simulink library "halout"  (R2021b)
settings: Solver=VariableStepAuto  StartTime=0.0  StopTime=10.0  RelTol=1e-3
undefined symbols (not defined in the file): C_TASK_5MS_S, FALSE, KHAL_CAN1FD1APS3E2E_flg, KHAL_CAN1FD1APS3TxReq_flg, KHAL_CAN1FD1VCU2E2E_flg, KHAL_CAN1FD1VCU2TxReq_flg, KHAL_CAN1FD1VCU3E2E_flg, KHAL_CAN1FD1VCU3TxReq_flg, KHAL_CAN1TxReq_flg, KHAL_CAN1VMCFCM1E2E_flg, KHAL_CAN1VMCFCM1TxReq_flg, KHAL_CAN2TxReq_flg, KHAL_CAN3FD3VCU1toNIDECTxReq_flg, KHAL_CAN3FD3VCU1TxReq_flg, KHAL_CAN3FD3VCU2E2E_flg, KHAL_CAN3FD3VCU2toNIDECE2E_flg, KHAL_CAN3FD3VCU2toNIDECTxReq_flg, KHAL_CAN3FD3VCU2TxReq_flg, KHAL_CAN3TxReq_flg, KHAL_CAN4FD4CE1000E2E_flg, KHAL_CAN4FD4CE1000TxReq_flg, KHAL_CAN4TxReq_flg, KHAL_CAN5TxReq_flg, KHAL_CAN6FD6APS3E2E_flg, KHAL_CAN6FD6APS3TxReq_flg, KHAL_CAN6FD6VCU2E2E_flg, KHAL_CAN6FD6VCU2TxReq_flg, KHAL_CAN6TxReq_flg, ONE_INT, TRUE, ZERO_INT
libraries: FVT_lib x549, simulink x244
(part 11 of 27)

== system halout/HAL_OUT/CAN4/FD4_CE100_0_Tx ==
  TxReq : Inport
  BSCP_outputs : Inport  Port=2  OutDataTypeStr=Bus: BSCP_outputs
  BOUTP_outputs : Inport  Port=3  OutDataTypeStr=Bus: BOUTP_outputs
  Chart : Stateflow chart  TreatAsAtomicUnit=on
  Constant : Constant  Value=C_TASK_5MS_S
  Constant3 : Constant  Value=CycleTime
  Data Type Conversion : DataTypeConversion  OutDataTypeStr=uint16
  Data Type Conversion1 : DataTypeConversion  OutDataTypeStr=uint8
  Divide : Product  Inputs=*/
  Gain : Gain  Gain=0.001
  Ground{,1..19} (20 alike) : Ground
  OR : Logic  Operator=OR  Inputs=77  AllPortsSameDT=off  OutDataTypeStr=boolean
  bus_selector : BusSelector  OutputSignals=VOUTP_APSStaSys_enum
  bus_selector1 : BusSelector  OutputSignals=VOUTP_AllDoorSW_flg
  bus_selector10 : BusSelector  OutputSignals=VOUTP_DKCAuthSta_enum
  bus_selector11 : BusSelector  OutputSignals=VOUTP_Dimmer_pct
  bus_selector12 : BusSelector  OutputSignals=VOUTP_DimmerEN_flg
  bus_selector13 : BusSelector  OutputSignals=VOUTP_DoorLockIND_flg
  bus_selector14 : BusSelector  OutputSignals=VOUTP_DrDoorSW_flg
  bus_selector15 : BusSelector  OutputSignals=VOUTP_DrSeatSta_enum
  bus_selector16 : BusSelector  OutputSignals=VOUTP_EquivAccPedalSWSta_flg
  bus_selector17 : BusSelector  OutputSignals=VOUTP_FrChargingDoorCtrl_enum
  bus_selector18 : BusSelector  OutputSignals=VOUTP_FrWiperH_flg
  bus_selector19 : BusSelector  OutputSignals=VOUTP_FrWiperL_flg
  bus_selector2 : BusSelector  OutputSignals=VOUTP_AntitheftSeatFlod_flg
  bus_selector20 : BusSelector  OutputSignals=VOUTP_HBeam_flg
  bus_selector21 : BusSelector  OutputSignals=VOUTP_HBeamADB_flg
  bus_selector22 : BusSelector  OutputSignals=VOUTP_HazardSW_flg
  bus_selector23 : BusSelector  OutputSignals=VOUTP_HoodSW_flg
  bus_selector24 : BusSelector  OutputSignals=VOUTP_HornCtrl_flg
  bus_selector25 : BusSelector  OutputSignals=VOUTP_LBSD_flg
  bus_selector26 : BusSelector  OutputSignals=VOUTP_LDRL_flg
  bus_selector27 : BusSelector  OutputSignals=VOUTP_LTurnLP_flg
  bus_selector28 : BusSelector  OutputSignals=VOUTP_LBeam_flg
  bus_selector29 : BusSelector  OutputSignals=VOUTP_LampPwr_flg
  bus_selector3 : BusSelector  OutputSignals=VOUTP_AntitheftSta_enum
  bus_selector30 : BusSelector  OutputSignals=VOUTP_LockSetting_flg
  bus_selector31 : BusSelector  OutputSignals=VOUTP_MSACtrlSta_enum
  bus_selector32 : BusSelector  OutputSignals=VOUTP_MirrorCtrl_enum
  bus_selector33 : BusSelector  OutputSignals=VOUTP_MirrorDefog_flg
  bus_selector34 : BusSelector  OutputSignals=VOUTP_PosLamp_flg
  bus_selector35 : BusSelector  OutputSignals=VOUTP_PsDoorSW_flg
  bus_selector36 : BusSelector  OutputSignals=VOUTP_PowerSta_enum
  bus_selector37 : BusSelector  OutputSignals=VOUTP_RBSD_flg
  bus_selector38 : BusSelector  OutputSignals=VOUTP_RDRL_flg
  bus_selector39 : BusSelector  OutputSignals=VOUTP_RLDoorSW_flg
  bus_selector4 : BusSelector  OutputSignals=VOUTP_BCMDoorLockSta_flg
  bus_selector40 : BusSelector  OutputSignals=VOUTP_RRDoorSW_flg
  bus_selector41 : BusSelector  OutputSignals=VOUTP_RTurnLP_flg
  bus_selector42 : BusSelector  OutputSignals=VOUTP_ReBrakeLPReq_flg
  bus_selector43 : BusSelector  OutputSignals=VOUTP_ReverseLamp_flg
  bus_selector44 : BusSelector  OutputSignals=VOUTP_RoomLampH_flg
  bus_selector45 : BusSelector  OutputSignals=VOUTP_RoomLampL_flg
  bus_selector46 : BusSelector  OutputSignals=VOUTP_RrChargingDoorCtrl_enum
  bus_selector47 : BusSelector  OutputSignals=VOUTP_RrDefog_flg
  bus_selector48 : BusSelector  OutputSignals=VOUTP_RrFogLamp_flg
  bus_selector49 : BusSelector  OutputSignals=VOUTP_RrWiper_flg
  bus_selector5 : BusSelector  OutputSignals=VOUTP_BrakeLamp_flg
  bus_selector50 : BusSelector  OutputSignals=VOUTP_ShiftGearPosn_enum
  bus_selector51 : BusSelector  OutputSignals=VOUTP_TailgateHDSW_flg
  bus_selector52 : BusSelector  OutputSignals=VOUTP_TailgateRemote_enum
  bus_selector53 : BusSelector  OutputSignals=VOUTP_TailgateSW_flg
  bus_selector54 : BusSelector  OutputSignals=VOUTP_TrunkRel_flg
  bus_selector55 : BusSelector  OutputSignals=VOUTP_WasherCtrl_enum
  bus_selector56 : BusSelector  OutputSignals=VOUTP_WiperFixMode_flg
  bus_selector6 : BusSelector  OutputSignals=VOUTP_CCCtrlSta_enum
  bus_selector7 : BusSelector  OutputSignals=VOUTP_CTDCtrl_enum
  bus_selector8 : BusSelector  OutputSignals=VOUTP_CTDLockSW_flg
  bus_selector9 : BusSelector  OutputSignals=VOUTP_CrashDetd_flg
  convert_out : FVT_lib/hal/convert_out  gain=1  offset=0
  detect_change{,1..56} (57 alike) : simulink/Logic and Bit Operations/Detect Change  vinit=0  OutDataTypeStr=boolean
  TriggerDataUpdate : Outport
  TriggerCallCDD : Outport  Port=2
  wires:
  Data Type Conversion/1 -> Chart/3(CycleCnt)
  TxReq/1 -> Chart/1(TxReq)
  [EventReq_flg] -> Chart/2(EventReq)
  Constant/1 -> Divide/2
  Divide/1 -> Data Type Conversion/1
  Gain/1 -> Divide/1
  Constant3/1 -> Gain/1
  BSCP_outputs/1 -> [BSCP_outputs]
  BOUTP_outputs/1 -> [BOUTP_outputs]
  OR/1 -> [EventReq_flg]
  detect_change/1 -> OR/1
  bus_selector/1 -> detect_change/1  "<VOUTP_APSStaSys_enum>"
  [BOUTP_outputs] -> bus_selector/1
  detect_change1/1 -> OR/2
  bus_selector1/1 -> detect_change1/1  "<VOUTP_AllDoorSW_flg>"
  [BOUTP_outputs] -> bus_selector1/1
  detect_change2/1 -> OR/3
  bus_selector2/1 -> detect_change2/1  "<VOUTP_AntitheftSeatFlod_flg>"
  [BOUTP_outputs] -> bus_selector2/1
  detect_change3/1 -> OR/4
  bus_selector3/1 -> detect_change3/1  "<VOUTP_AntitheftSta_enum>"
  [BOUTP_outputs] -> bus_selector3/1
  detect_change4/1 -> OR/5
  bus_selector4/1 -> detect_change4/1  "<VOUTP_BCMDoorLockSta_flg>"
  [BOUTP_outputs] -> bus_selector4/1
  detect_change5/1 -> OR/6
  bus_selector5/1 -> detect_change5/1  "<VOUTP_BrakeLamp_flg>"
  [BOUTP_outputs] -> bus_selector5/1
  detect_change6/1 -> OR/7
  bus_selector6/1 -> detect_change6/1  "<VOUTP_CCCtrlSta_enum>"
  [BOUTP_outputs] -> bus_selector6/1
  Ground/1 -> OR/8
  detect_change7/1 -> OR/9
  bus_selector7/1 -> detect_change7/1  "<VOUTP_CTDCtrl_enum>"
  [BOUTP_outputs] -> bus_selector7/1
  detect_change8/1 -> OR/10
  bus_selector8/1 -> detect_change8/1  "<VOUTP_CTDLockSW_flg>"
  [BOUTP_outputs] -> bus_selector8/1
  Ground1/1 -> OR/11
  detect_change9/1 -> OR/12
  bus_selector9/1 -> detect_change9/1  "<VOUTP_CrashDetd_flg>"
  [BOUTP_outputs] -> bus_selector9/1
  Ground2/1 -> OR/13
  Ground3/1 -> OR/14
  Ground4/1 -> OR/15
  Ground5/1 -> OR/16
  Ground6/1 -> OR/17
  detect_change10/1 -> OR/18
  bus_selector10/1 -> detect_change10/1  "<VOUTP_DKCAuthSta_enum>"
  [BOUTP_outputs] -> bus_selector10/1
  Ground7/1 -> OR/19
  detect_change11/1 -> OR/20
  Data Type Conversion1/1 -> detect_change11/1
  convert_out/1 -> Data Type Conversion1/1
  bus_selector11/1 -> convert_out/1  "<VOUTP_Dimmer_pct>"
  [BOUTP_outputs] -> bus_selector11/1
  detect_change12/1 -> OR/21
  bus_selector12/1 -> detect_change12/1  "<VOUTP_DimmerEN_flg>"
  [BOUTP_outputs] -> bus_selector12/1
  detect_change13/1 -> OR/22
  bus_selector13/1 -> detect_change13/1  "<VOUTP_DoorLockIND_flg>"
  [BOUTP_outputs] -> bus_selector13/1
  detect_change14/1 -> OR/23
  bus_selector14/1 -> detect_change14/1  "<VOUTP_DrDoorSW_flg>"
  [BOUTP_outputs] -> bus_selector14/1
  detect_change15/1 -> OR/24
  bus_selector15/1 -> detect_change15/1  "<VOUTP_DrSeatSta_enum>"
  [BOUTP_outputs] -> bus_selector15/1
  detect_change16/1 -> OR/25
  bus_selector16/1 -> detect_change16/1  "<VOUTP_EquivAccPedalSWSta_flg>"
  [BOUTP_outputs] -> bus_selector16/1
  Ground8/1 -> OR/26
  Ground9/1 -> OR/27
  Ground10/1 -> OR/28
  Ground11/1 -> OR/29
  Ground12/1 -> OR/30
  Ground13/1 -> OR/31
  Ground14/1 -> OR/32
  detect_change17/1 -> OR/33
  bus_selector17/1 -> detect_change17/1  "<VOUTP_FrChargingDoorCtrl_enum>"
  [BOUTP_outputs] -> bus_selector17/1
  Ground15/1 -> OR/34
  detect_change18/1 -> OR/35
  bus_selector18/1 -> detect_change18/1  "<VOUTP_FrWiperH_flg>"
  [BOUTP_outputs] -> bus_selector18/1
  detect_change19/1 -> OR/36
  bus_selector19/1 -> detect_change19/1  "<VOUTP_FrWiperL_flg>"
  [BOUTP_outputs] -> bus_selector19/1
  Ground16/1 -> OR/37
  detect_change20/1 -> OR/38
  bus_selector20/1 -> detect_change20/1  "<VOUTP_HBeam_flg>"
  [BOUTP_outputs] -> bus_selector20/1
  detect_change21/1 -> OR/39
  bus_selector21/1 -> detect_change21/1  "<VOUTP_HBeamADB_flg>"
  [BOUTP_outputs] -> bus_selector21/1
  detect_change22/1 -> OR/40
  bus_selector22/1 -> detect_change22/1  "<VOUTP_HazardSW_flg>"
  [BOUTP_outputs] -> bus_selector22/1
  detect_change23/1 -> OR/41
  bus_selector23/1 -> detect_change23/1  "<VOUTP_HoodSW_flg>"
  [BOUTP_outputs] -> bus_selector23/1
  detect_change24/1 -> OR/42
  bus_selector24/1 -> detect_change24/1  "<VOUTP_HornCtrl_flg>"
  [BOUTP_outputs] -> bus_selector24/1
  detect_change25/1 -> OR/43
  bus_selector25/1 -> detect_change25/1  "<VOUTP_LBSD_flg>"
  [BOUTP_outputs] -> bus_selector25/1
  detect_change26/1 -> OR/44
  bus_selector26/1 -> detect_change26/1  "<VOUTP_LDRL_flg>"
  [BOUTP_outputs] -> bus_selector26/1
  detect_change27/1 -> OR/45
  bus_selector27/1 -> detect_change27/1  "<VOUTP_LTurnLP_flg>"
  [BOUTP_outputs] -> bus_selector27/1
  Ground17/1 -> OR/46
  detect_change28/1 -> OR/47
  bus_selector28/1 -> detect_change28/1  "<VOUTP_LBeam_flg>"
  [BOUTP_outputs] -> bus_selector28/1
  detect_change29/1 -> OR/48
  bus_selector29/1 -> detect_change29/1  "<VOUTP_LampPwr_flg>"
  [BOUTP_outputs] -> bus_selector29/1
  detect_change30/1 -> OR/49
  bus_selector30/1 -> detect_change30/1  "<VOUTP_LockSetting_flg>"
  [BOUTP_outputs] -> bus_selector30/1
  detect_change31/1 -> OR/50
  bus_selector31/1 -> detect_change31/1  "<VOUTP_MSACtrlSta_enum>"
  [BOUTP_outputs] -> bus_selector31/1
  detect_change32/1 -> OR/51
  bus_selector32/1 -> detect_change32/1  "<VOUTP_MirrorCtrl_enum>"
  [BOUTP_outputs] -> bus_selector32/1
  detect_change33/1 -> OR/52
  bus_selector33/1 -> detect_change33/1  "<VOUTP_MirrorDefog_flg>"
  [BOUTP_outputs] -> bus_selector33/1
  detect_change34/1 -> OR/53
  bus_selector34/1 -> detect_change34/1  "<VOUTP_PosLamp_flg>"
  [BOUTP_outputs] -> bus_selector34/1
  detect_change35/1 -> OR/54
  bus_selector35/1 -> detect_change35/1  "<VOUTP_PsDoorSW_flg>"
  [BOUTP_outputs] -> bus_selector35/1
  detect_change36/1 -> OR/55
  bus_selector36/1 -> detect_change36/1  "<VOUTP_PowerSta_enum>"
  [BOUTP_outputs] -> bus_selector36/1
  detect_change37/1 -> OR/56
  bus_selector37/1 -> detect_change37/1  "<VOUTP_RBSD_flg>"
  [BOUTP_outputs] -> bus_selector37/1
  Ground18/1 -> OR/57
  detect_change38/1 -> OR/58
  bus_selector38/1 -> detect_change38/1  "<VOUTP_RDRL_flg>"
  [BOUTP_outputs] -> bus_selector38/1
  detect_change39/1 -> OR/59
  bus_selector39/1 -> detect_change39/1  "<VOUTP_RLDoorSW_flg>"
  [BOUTP_outputs] -> bus_selector39/1
  detect_change40/1 -> OR/60
  bus_selector40/1 -> detect_change40/1  "<VOUTP_RRDoorSW_flg>"
  [BOUTP_outputs] -> bus_selector40/1
  detect_change41/1 -> OR/61
  bus_selector41/1 -> detect_change41/1  "<VOUTP_RTurnLP_flg>"
  [BOUTP_outputs] -> bus_selector41/1
  detect_change42/1 -> OR/62
  bus_selector42/1 -> detect_change42/1  "<VOUTP_ReBrakeLPReq_flg>"
  [BOUTP_outputs] -> bus_selector42/1
  detect_change43/1 -> OR/63
  bus_selector43/1 -> detect_change43/1  "<VOUTP_ReverseLamp_flg>"
  [BOUTP_outputs] -> bus_selector43/1
  detect_change44/1 -> OR/64
  bus_selector44/1 -> detect_change44/1  "<VOUTP_RoomLampH_flg>"
  [BOUTP_outputs] -> bus_selector44/1
  detect_change45/1 -> OR/65
  bus_selector45/1 -> detect_change45/1  "<VOUTP_RoomLampL_flg>"
  [BOUTP_outputs] -> bus_selector45/1
  detect_change46/1 -> OR/66
  bus_selector46/1 -> detect_change46/1  "<VOUTP_RrChargingDoorCtrl_enum>"
  [BOUTP_outputs] -> bus_selector46/1
  detect_change47/1 -> OR/67
  bus_selector47/1 -> detect_change47/1  "<VOUTP_RrDefog_flg>"
  [BOUTP_outputs] -> bus_selector47/1
  detect_change48/1 -> OR/68
  bus_selector48/1 -> detect_change48/1  "<VOUTP_RrFogLamp_flg>"
  [BOUTP_outputs] -> bus_selector48/1
  detect_change49/1 -> OR/69
  bus_selector49/1 -> detect_change49/1  "<VOUTP_RrWiper_flg>"
  [BOUTP_outputs] -> bus_selector49/1
  detect_change50/1 -> OR/70
  bus_selector50/1 -> detect_change50/1  "<VOUTP_ShiftGearPosn_enum>"
  [BOUTP_outputs] -> bus_selector50/1
  detect_change51/1 -> OR/71
  bus_selector51/1 -> detect_change51/1  "<VOUTP_TailgateHDSW_flg>"
  [BOUTP_outputs] -> bus_selector51/1
  detect_change52/1 -> OR/72
  bus_selector52/1 -> detect_change52/1  "<VOUTP_TailgateRemote_enum>"
  [BOUTP_outputs] -> bus_selector52/1
  detect_change53/1 -> OR/73
  bus_selector53/1 -> detect_change53/1  "<VOUTP_TailgateSW_flg>"
  [BOUTP_outputs] -> bus_selector53/1
  Ground19/1 -> OR/74
  detect_change54/1 -> OR/75
  bus_selector54/1 -> detect_change54/1  "<VOUTP_TrunkRel_flg>"
  [BOUTP_outputs] -> bus_selector54/1
  detect_change55/1 -> OR/76
  bus_selector55/1 -> detect_change55/1  "<VOUTP_WasherCtrl_enum>"
  [BOUTP_outputs] -> bus_selector55/1
  detect_change56/1 -> OR/77
  bus_selector56/1 -> detect_change56/1  "<VOUTP_WiperFixMode_flg>"
  [BOUTP_outputs] -> bus_selector56/1
  Chart/1(TriggerDataUpdate()) -> TriggerDataUpdate/1
  Chart/2(TriggerCallCDD()) -> TriggerCallCDD/1

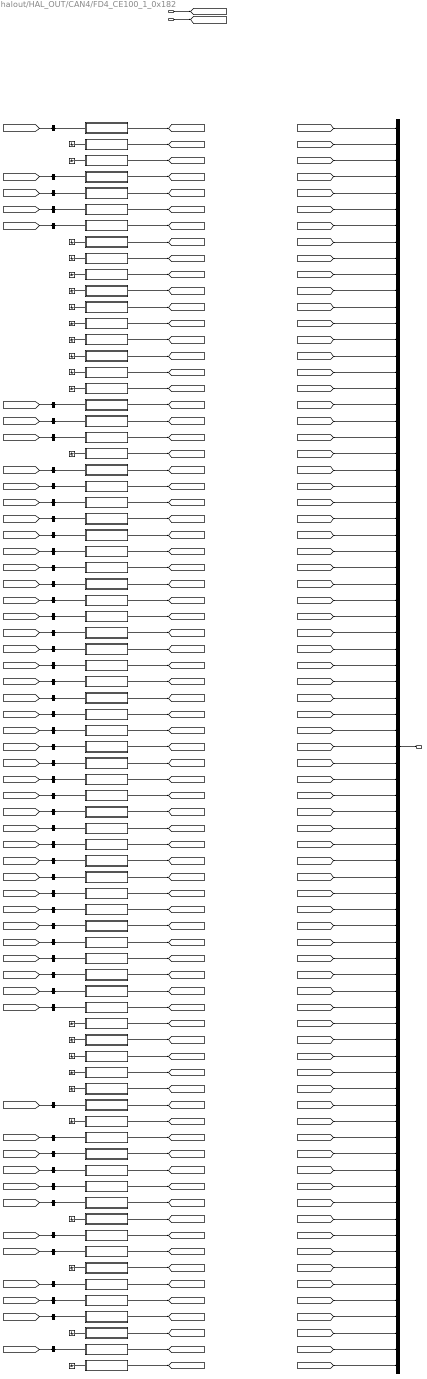
== system halout/HAL_OUT/CAN4/FD4_CE100_1_0x182 ==
  BSCP_outputs : Inport  OutDataTypeStr=Bus: BSCP_outputs
  BOUTP_outputs : Inport  Port=2  OutDataTypeStr=Bus: BOUTP_outputs
  ACSubMode : Subsystem
  APTCActFrRiPwr : Subsystem
  BatLoopActWtFlw : Subsystem
  BatteryMode : Subsystem
  CCUACLampSts : Subsystem
  CCUACMaxLampSts : Subsystem
  CCUAutoLampSts : Subsystem
  CCUAutoMidLampSts : Subsystem
  CCUCbnPreACWkSts : Subsystem
  CCUCbnPreEstimdTi : Subsystem
  CCUCbnPreSts : Subsystem
  CCUDispalyRequest : Subsystem
  CCUEcoSts : Subsystem
  CCUFrtOnOffLampSts : Subsystem
  CCUHEATMaxLampSts : Subsystem
  CCUHiVoltageReq : Subsystem
  CCURrOnOffLampSts : Subsystem
  CCUSyncLampSts : Subsystem
  CabinMode : Subsystem
  CoolgFanActDuty : Subsystem
  DeiceModReq : Subsystem
  EDriveMode : Subsystem
  FDAGSCmd : Subsystem
  FDBlowerCmd : Subsystem
  FDCTHCMCLEVentYSta : Subsystem
  FDCTHCMCLEVentZSta : Subsystem
  FDCTHCMCLVentSta : Subsystem
  FDCTHCMCREVentYSta : Subsystem
  FDCTHCMCREVentZSta : Subsystem
  FDCTHCMCRVentSta : Subsystem
  FDCTHCMDrEVentModeSta : Subsystem
  FDCTHCMDrEVentYSta : Subsystem
  FDCTHCMDrEVentZSta : Subsystem
  FDCTHCMDrVentSta : Subsystem
  FDCTHCMPsEVentModeSta : Subsystem
  FDCTHCMPsEVentYSta : Subsystem
  FDCTHCMPsEVentZSta : Subsystem
  FDCTHCMPsVentSta : Subsystem
  FDCompCmd : Subsystem
  FDEWP1Cmd : Subsystem
  FDEWP2Cmd : Subsystem
  FDEWP3Cmd : Subsystem
  FDEXV1Cmd : Subsystem
  FDEXV2Cmd : Subsystem
  FDFWVCmd : Subsystem
  FDFrLeAPTCHeatPwrCmd : Subsystem
  FDFrRiAPTCHeatPwrCmd : Subsystem
  FDFrWPTCHeatPwrCmd : Subsystem
  FDRecyAutoCmd : Subsystem
  FDRrAPTCHeatPwrCmd : Subsystem
  FDSOTXVCmd : Subsystem
  FDSOV1Cmd : Subsystem
  FDSOV2Cmd : Subsystem
  FDSOV3Cmd : Subsystem
  FDTWVCmd : Subsystem
  FrCoolantflow : Subsystem
  FrCoolanttemp : Subsystem
  Ground{,1..18,20..23} (23 alike) : Ground
  HPThermalRecoveryReq : Subsystem
  RrCoolantflow : Subsystem
  RrCoolanttemp : Subsystem
  bus_creator : BusCreator  Inputs=77  OutDataTypeStr=Bus: DT_CAN4_SG_FD4_CE100_1  NonVirtualBus=on
  bus_selector : BusSelector  OutputSignals=VOUTP_ACSubMode_enum
  bus_selector1 : BusSelector  OutputSignals=VOUTP_BatteryMode_enum
  bus_selector10 : BusSelector  OutputSignals=VOUTP_FDCTHCCLEVentZSta_enum
  bus_selector11 : BusSelector  OutputSignals=VOUTP_FDCTHCCLVentENSta_flg
  bus_selector12 : BusSelector  OutputSignals=VOUTP_FDCTHCCREVentYSta_enum
  bus_selector13 : BusSelector  OutputSignals=VOUTP_FDCTHCCREVentZSta_enum
  bus_selector14 : BusSelector  OutputSignals=VOUTP_FDCTHCLEVentModeSta_enum
  bus_selector15 : BusSelector  OutputSignals=VOUTP_FDCTHCLEVentYSta_enum
  bus_selector16 : BusSelector  OutputSignals=VOUTP_FDCTHCLEVentZSta_enum
  bus_selector17 : BusSelector  OutputSignals=VOUTP_FDCTHCRVentENSta_flg
  bus_selector18 : BusSelector  OutputSignals=VOUTP_FDCTHCLVentENSta_flg
  bus_selector19 : BusSelector  OutputSignals=VOUTP_FDCTHCREVentModeSta_enum
  bus_selector2 : BusSelector  OutputSignals=VOUTP_CCUACLampSts_flg
  bus_selector20 : BusSelector  OutputSignals=VOUTP_FDCTHCREVentYSta_enum
  bus_selector21 : BusSelector  OutputSignals=VOUTP_FDCTHCREVentZSta_enum
  bus_selector22 : BusSelector  OutputSignals=VOUTP_FDCTHCRVentENSta_flg
  bus_selector23 : BusSelector  OutputSignals=VOUTP_FDAGSCmd_enum
  bus_selector24 : BusSelector  OutputSignals=VOUTP_FDBlowerCmd_pct
  bus_selector25 : BusSelector  OutputSignals=VOUTP_FDCompCmd_rpm
  bus_selector26 : BusSelector  OutputSignals=VOUTP_FDEWP1Cmd_enum
  bus_selector27 : BusSelector  OutputSignals=VOUTP_FDEWP2Cmd_enum
  bus_selector28 : BusSelector  OutputSignals=VOUTP_FDEWP3Cmd_enum
  bus_selector29 : BusSelector  OutputSignals=VOUTP_FDEXV1Cmd_step
  bus_selector3 : BusSelector  OutputSignals=VOUTP_CCUACMaxLampSts_flg
  bus_selector30 : BusSelector  OutputSignals=VOUTP_FDEXV2Cmd_step
  bus_selector31 : BusSelector  OutputSignals=VOUTP_FDFWVCmd_flg
  bus_selector32 : BusSelector  OutputSignals=VOUTP_FDFrLeAPTCHeatPwrCmd_W
  bus_selector33 : BusSelector  OutputSignals=VOUTP_FDFrRiAPTCHeatPwrCmd_W
  bus_selector34 : BusSelector  OutputSignals=VOUTP_FDFrWPTCHeatPwrCmd_W
  bus_selector35 : BusSelector  OutputSignals=VOUTP_FDRecyAutoCmd_enum
  bus_selector36 : BusSelector  OutputSignals=VOUTP_FDRrAPTCHeatPwrCmd_W
  bus_selector37 : BusSelector  OutputSignals=VOUTP_FDSOTXVCmd_flg
  bus_selector38 : BusSelector  OutputSignals=VOUTP_FDSOV1Cmd_flg
  bus_selector39 : BusSelector  OutputSignals=VOUTP_FDSOV2Cmd_flg
  bus_selector4 : BusSelector  OutputSignals=VOUTP_CCUAutoLampSts_flg
  bus_selector40 : BusSelector  OutputSignals=VOUTP_FDSOV3Cmd_flg
  bus_selector41 : BusSelector  OutputSignals=VOUTP_FDTWVCmd_pct
  bus_selector42 : BusSelector  OutputSignals=VOUTP_sigAirIntenZon1St_enum
  bus_selector43 : BusSelector  OutputSignals=VOUTP_sigAmbAirT_C
  bus_selector44 : BusSelector  OutputSignals=VOUTP_sigCbnAirT_C
  bus_selector45 : BusSelector  OutputSignals=VOUTP_sigCbnSolarLeft_W
  bus_selector46 : BusSelector  OutputSignals=VOUTP_sigCbnSolarRight_W
  bus_selector47 : BusSelector  OutputSignals=VOUTP_sigClntTHvBattOut_C
  bus_selector48 : BusSelector  OutputSignals=VOUTP_sigDfrstSt_flg
  bus_selector49 : BusSelector  OutputSignals=VOUTP_sigRecircSt_flg
  bus_selector5 : BusSelector  OutputSignals=VOUTP_CCUSyncLampSts_flg
  bus_selector50 : BusSelector  OutputSignals=VOUTP_sigSetTempZon1St_C
  bus_selector51 : BusSelector  OutputSignals=VOUTP_sigSetTempZon2St_C
  bus_selector52 : BusSelector  OutputSignals=VOUTP_sigWindDirZon1St_enum
  bus_selector53 : BusSelector  OutputSignals=VOUTP_sigCbnPTCPwrAct_W
  bus_selector6 : BusSelector  OutputSignals=VOUTP_CabinMode_enum
  bus_selector7 : BusSelector  OutputSignals=VOUTP_CoolgFanActDuty_pct
  bus_selector8 : BusSelector  OutputSignals=VOUTP_EDriveMode_enum
  bus_selector9 : BusSelector  OutputSignals=VOUTP_FDCTHCCLEVentYSta_enum
  sigAirIntenZon1St : Subsystem
  sigAirIntenZon3St : Subsystem
  sigAmbAirT : Subsystem
  sigCbnAirT : Subsystem
  sigCbnPTCPwrAct : Subsystem
  sigCbnSolarLeft : Subsystem
  sigCbnSolarRight : Subsystem
  sigClmtCmprPwrAct : Subsystem
  sigClntTHvBattOut : Subsystem
  sigDfrstSt : Subsystem
  sigHvacSt : Subsystem
  sigRecircSt : Subsystem
  sigSetTempZon1St : Subsystem
  sigSetTempZon2St : Subsystem
  sigSetTempZon3St : Subsystem
  sigWindDirZon1St : Subsystem
  sigWindDirZon3St : Subsystem
  FD4_CE100_1 : Outport
  wires:
  BSCP_outputs/1 -> [BSCP_outputs]
  BOUTP_outputs/1 -> [BOUTP_outputs]
  [CAN4_ACSubMode] -> bus_creator/1  "CAN4_ACSubMode"
  [CAN4_APTC_ActFrRiPwr] -> bus_creator/2  "CAN4_APTC_ActFrRiPwr"
  [CAN4_BatLoopActWtFlw] -> bus_creator/3  "CAN4_BatLoopActWtFlw"
  [CAN4_BatteryMode] -> bus_creator/4  "CAN4_BatteryMode"
  [CAN4_CCU_ACLampSts] -> bus_creator/5  "CAN4_CCU_ACLampSts"
  [CAN4_CCU_ACMaxLampSts] -> bus_creator/6  "CAN4_CCU_ACMaxLampSts"
  [CAN4_CCU_AutoLampSts] -> bus_creator/7  "CAN4_CCU_AutoLampSts"
  [CAN4_CCU_AutoMidLampSts] -> bus_creator/8  "CAN4_CCU_AutoMidLampSts"
  [CAN4_CCU_CbnPreACWkSts] -> bus_creator/9  "CAN4_CCU_CbnPreACWkSts"
  [CAN4_CCU_CbnPreEstimdTi] -> bus_creator/10  "CAN4_CCU_CbnPreEstimdTi"
  [CAN4_CCU_CbnPreSts] -> bus_creator/11  "CAN4_CCU_CbnPreSts"
  [CAN4_CCU_Dispaly_Request] -> bus_creator/12  "CAN4_CCU_Dispaly_Request"
  [CAN4_CCU_EcoSts] -> bus_creator/13  "CAN4_CCU_EcoSts"
  [CAN4_CCU_FrtOnOffLampSts] -> bus_creator/14  "CAN4_CCU_FrtOnOffLampSts"
  [CAN4_CCU_HEATMaxLampSts] -> bus_creator/15  "CAN4_CCU_HEATMaxLampSts"
  [CAN4_CCU_HiVoltageReq] -> bus_creator/16  "CAN4_CCU_HiVoltageReq"
  [CAN4_CCU_RrOnOffLampSts] -> bus_creator/17  "CAN4_CCU_RrOnOffLampSts"
  [CAN4_CCU_SyncLampSts] -> bus_creator/18  "CAN4_CCU_SyncLampSts"
  [CAN4_CabinMode] -> bus_creator/19  "CAN4_CabinMode"
  [CAN4_CoolgFanActDuty] -> bus_creator/20  "CAN4_CoolgFanActDuty"
  [CAN4_DeiceModReq] -> bus_creator/21  "CAN4_DeiceModReq"
  [CAN4_EDriveMode] -> bus_creator/22  "CAN4_EDriveMode"
  [CAN4_FDC_THCM_CLEVentY_Sta] -> bus_creator/23  "CAN4_FDC_THCM_CLEVentY_Sta"
  [CAN4_FDC_THCM_CLEVentZ_Sta] -> bus_creator/24  "CAN4_FDC_THCM_CLEVentZ_Sta"
  [CAN4_FDC_THCM_CLVent_Sta] -> bus_creator/25  "CAN4_FDC_THCM_CLVent_Sta"
  [CAN4_FDC_THCM_CREVentY_Sta] -> bus_creator/26  "CAN4_FDC_THCM_CREVentY_Sta"
  [CAN4_FDC_THCM_CREVentZ_Sta] -> bus_creator/27  "CAN4_FDC_THCM_CREVentZ_Sta"
  [CAN4_FDC_THCM_CRVent_Sta] -> bus_creator/28  "CAN4_FDC_THCM_CRVent_Sta"
  [CAN4_FDC_THCM_DrEVentMode_Sta] -> bus_creator/29  "CAN4_FDC_THCM_DrEVentMode_Sta"
  [CAN4_FDC_THCM_DrEVentY_Sta] -> bus_creator/30  "CAN4_FDC_THCM_DrEVentY_Sta"
  [CAN4_FDC_THCM_DrEVentZ_Sta] -> bus_creator/31  "CAN4_FDC_THCM_DrEVentZ_Sta"
  [CAN4_FDC_THCM_DrVent_Sta] -> bus_creator/32  "CAN4_FDC_THCM_DrVent_Sta"
  [CAN4_FDC_THCM_PsEVentMode_Sta] -> bus_creator/33  "CAN4_FDC_THCM_PsEVentMode_Sta"
  [CAN4_FDC_THCM_PsEVentY_Sta] -> bus_creator/34  "CAN4_FDC_THCM_PsEVentY_Sta"
  [CAN4_FDC_THCM_PsEVentZ_Sta] -> bus_creator/35  "CAN4_FDC_THCM_PsEVentZ_Sta"
  [CAN4_FDC_THCM_PsVent_Sta] -> bus_creator/36  "CAN4_FDC_THCM_PsVent_Sta"
  [CAN4_FD_AGS_Cmd] -> bus_creator/37  "CAN4_FD_AGS_Cmd"
  [CAN4_FD_Blower_Cmd] -> bus_creator/38  "CAN4_FD_Blower_Cmd"
  [CAN4_FD_Comp_Cmd] -> bus_creator/39  "CAN4_FD_Comp_Cmd"
  [CAN4_FD_EWP1_Cmd] -> bus_creator/40  "CAN4_FD_EWP1_Cmd"
  [CAN4_FD_EWP2_Cmd] -> bus_creator/41  "CAN4_FD_EWP2_Cmd"
  [CAN4_FD_EWP3_Cmd] -> bus_creator/42  "CAN4_FD_EWP3_Cmd"
  [CAN4_FD_EXV1_Cmd] -> bus_creator/43  "CAN4_FD_EXV1_Cmd"
  [CAN4_FD_EXV2_Cmd] -> bus_creator/44  "CAN4_FD_EXV2_Cmd"
  [CAN4_FD_FWV_Cmd] -> bus_creator/45  "CAN4_FD_FWV_Cmd"
  [CAN4_FD_FrLeAPTCHeatPwr_Cmd] -> bus_creator/46  "CAN4_FD_FrLeAPTCHeatPwr_Cmd"
  [CAN4_FD_FrRiAPTCHeatPwr_Cmd] -> bus_creator/47  "CAN4_FD_FrRiAPTCHeatPwr_Cmd"
  [CAN4_FD_FrWPTCHeatPwr_Cmd] -> bus_creator/48  "CAN4_FD_FrWPTCHeatPwr_Cmd"
  [CAN4_FD_RecyAuto_Cmd] -> bus_creator/49  "CAN4_FD_RecyAuto_Cmd"
  [CAN4_FD_RrAPTCHeatPwr_Cmd] -> bus_creator/50  "CAN4_FD_RrAPTCHeatPwr_Cmd"
  [CAN4_FD_SOTXV_Cmd] -> bus_creator/51  "CAN4_FD_SOTXV_Cmd"
  [CAN4_FD_SOV1_Cmd] -> bus_creator/52  "CAN4_FD_SOV1_Cmd"
  [CAN4_FD_SOV2_Cmd] -> bus_creator/53  "CAN4_FD_SOV2_Cmd"
  [CAN4_FD_SOV3_Cmd] -> bus_creator/54  "CAN4_FD_SOV3_Cmd"
  [CAN4_FD_TWV_Cmd] -> bus_creator/55  "CAN4_FD_TWV_Cmd"
  [CAN4_Fr_Coolantflow] -> bus_creator/56  "CAN4_Fr_Coolantflow"
  [CAN4_Fr_Coolanttemp] -> bus_creator/57  "CAN4_Fr_Coolanttemp"
  [CAN4_HPThermalRecoveryReq] -> bus_creator/58  "CAN4_HPThermalRecoveryReq"
  [CAN4_Rr_Coolantflow] -> bus_creator/59  "CAN4_Rr_Coolantflow"
  [CAN4_Rr_Coolanttemp] -> bus_creator/60  "CAN4_Rr_Coolanttemp"
  [CAN4_sigAirIntenZon1St] -> bus_creator/61  "CAN4_sigAirIntenZon1St"
  [CAN4_sigAirIntenZon3St] -> bus_creator/62  "CAN4_sigAirIntenZon3St"
  [CAN4_sigAmbAirT] -> bus_creator/63  "CAN4_sigAmbAirT"
  [CAN4_sigCbnAirT] -> bus_creator/64  "CAN4_sigCbnAirT"
  [CAN4_sigCbnPTCPwrAct] -> bus_creator/65  "CAN4_sigCbnPTCPwrAct"
  [CAN4_sigCbnSolarLeft] -> bus_creator/66  "CAN4_sigCbnSolarLeft"
  [CAN4_sigCbnSolarRight] -> bus_creator/67  "CAN4_sigCbnSolarRight"
  [CAN4_sigClmtCmprPwrAct] -> bus_creator/68  "CAN4_sigClmtCmprPwrAct"
  [CAN4_sigClntTHvBattOut] -> bus_creator/69  "CAN4_sigClntTHvBattOut"
  [CAN4_sigDfrstSt] -> bus_creator/70  "CAN4_sigDfrstSt"
  [CAN4_sigHvacSt] -> bus_creator/71  "CAN4_sigHvacSt"
  [CAN4_sigRecircSt] -> bus_creator/72  "CAN4_sigRecircSt"
  [CAN4_sigSetTempZon1St] -> bus_creator/73  "CAN4_sigSetTempZon1St"
  [CAN4_sigSetTempZon2St] -> bus_creator/74  "CAN4_sigSetTempZon2St"
  [CAN4_sigSetTempZon3St] -> bus_creator/75  "CAN4_sigSetTempZon3St"
  [CAN4_sigWindDirZon1St] -> bus_creator/76  "CAN4_sigWindDirZon1St"
  [CAN4_sigWindDirZon3St] -> bus_creator/77  "CAN4_sigWindDirZon3St"
  bus_creator/1 -> FD4_CE100_1/1
  ACSubMode/1(CAN4_ACSubMode) -> [CAN4_ACSubMode]
  APTCActFrRiPwr/1(CAN4_APTC_ActFrRiPwr) -> [CAN4_APTC_ActFrRiPwr]
  BatLoopActWtFlw/1(CAN4_BatLoopActWtFlw) -> [CAN4_BatLoopActWtFlw]
  BatteryMode/1(CAN4_BatteryMode) -> [CAN4_BatteryMode]
  CCUACLampSts/1(CAN4_CCU_ACLampSts) -> [CAN4_CCU_ACLampSts]
  CCUACMaxLampSts/1(CAN4_CCU_ACMaxLampSts) -> [CAN4_CCU_ACMaxLampSts]
  CCUAutoLampSts/1(CAN4_CCU_AutoLampSts) -> [CAN4_CCU_AutoLampSts]
  CCUAutoMidLampSts/1(CAN4_CCU_AutoMidLampSts) -> [CAN4_CCU_AutoMidLampSts]
  CCUCbnPreACWkSts/1(CAN4_CCU_CbnPreACWkSts) -> [CAN4_CCU_CbnPreACWkSts]
  CCUCbnPreEstimdTi/1(CAN4_CCU_CbnPreEstimdTi) -> [CAN4_CCU_CbnPreEstimdTi]
  CCUCbnPreSts/1(CAN4_CCU_CbnPreSts) -> [CAN4_CCU_CbnPreSts]
  CCUDispalyRequest/1(CAN4_CCU_Dispaly_Request) -> [CAN4_CCU_Dispaly_Request]
  CCUEcoSts/1(CAN4_CCU_EcoSts) -> [CAN4_CCU_EcoSts]
  CCUFrtOnOffLampSts/1(CAN4_CCU_FrtOnOffLampSts) -> [CAN4_CCU_FrtOnOffLampSts]
  CCUHEATMaxLampSts/1(CAN4_CCU_HEATMaxLampSts) -> [CAN4_CCU_HEATMaxLampSts]
  CCUHiVoltageReq/1(CAN4_CCU_HiVoltageReq) -> [CAN4_CCU_HiVoltageReq]
  CCURrOnOffLampSts/1(CAN4_CCU_RrOnOffLampSts) -> [CAN4_CCU_RrOnOffLampSts]
  CCUSyncLampSts/1(CAN4_CCU_SyncLampSts) -> [CAN4_CCU_SyncLampSts]
  CabinMode/1(CAN4_CabinMode) -> [CAN4_CabinMode]
  CoolgFanActDuty/1(CAN4_CoolgFanActDuty) -> [CAN4_CoolgFanActDuty]
  DeiceModReq/1(CAN4_DeiceModReq) -> [CAN4_DeiceModReq]
  EDriveMode/1(CAN4_EDriveMode) -> [CAN4_EDriveMode]
  FDCTHCMCLEVentYSta/1(CAN4_FDC_THCM_CLEVentY_Sta) -> [CAN4_FDC_THCM_CLEVentY_Sta]
  FDCTHCMCLEVentZSta/1(CAN4_FDC_THCM_CLEVentZ_Sta) -> [CAN4_FDC_THCM_CLEVentZ_Sta]
  FDCTHCMCLVentSta/1(CAN4_FDC_THCM_CLVent_Sta) -> [CAN4_FDC_THCM_CLVent_Sta]
  FDCTHCMCREVentYSta/1(CAN4_FDC_THCM_CREVentY_Sta) -> [CAN4_FDC_THCM_CREVentY_Sta]
  FDCTHCMCREVentZSta/1(CAN4_FDC_THCM_CREVentZ_Sta) -> [CAN4_FDC_THCM_CREVentZ_Sta]
  FDCTHCMCRVentSta/1(CAN4_FDC_THCM_CRVent_Sta) -> [CAN4_FDC_THCM_CRVent_Sta]
  FDCTHCMDrEVentModeSta/1(CAN4_FDC_THCM_DrEVentMode_Sta) -> [CAN4_FDC_THCM_DrEVentMode_Sta]
  FDCTHCMDrEVentYSta/1(CAN4_FDC_THCM_DrEVentY_Sta) -> [CAN4_FDC_THCM_DrEVentY_Sta]
  FDCTHCMDrEVentZSta/1(CAN4_FDC_THCM_DrEVentZ_Sta) -> [CAN4_FDC_THCM_DrEVentZ_Sta]
  FDCTHCMDrVentSta/1(CAN4_FDC_THCM_DrVent_Sta) -> [CAN4_FDC_THCM_DrVent_Sta]
  FDCTHCMPsEVentModeSta/1(CAN4_FDC_THCM_PsEVentMode_Sta) -> [CAN4_FDC_THCM_PsEVentMode_Sta]
  FDCTHCMPsEVentYSta/1(CAN4_FDC_THCM_PsEVentY_Sta) -> [CAN4_FDC_THCM_PsEVentY_Sta]
  FDCTHCMPsEVentZSta/1(CAN4_FDC_THCM_PsEVentZ_Sta) -> [CAN4_FDC_THCM_PsEVentZ_Sta]
  FDCTHCMPsVentSta/1(CAN4_FDC_THCM_PsVent_Sta) -> [CAN4_FDC_THCM_PsVent_Sta]
  FDAGSCmd/1(CAN4_FD_AGS_Cmd) -> [CAN4_FD_AGS_Cmd]
  FDBlowerCmd/1(CAN4_FD_Blower_Cmd) -> [CAN4_FD_Blower_Cmd]
  FDCompCmd/1(CAN4_FD_Comp_Cmd) -> [CAN4_FD_Comp_Cmd]
  FDEWP1Cmd/1(CAN4_FD_EWP1_Cmd) -> [CAN4_FD_EWP1_Cmd]
  FDEWP2Cmd/1(CAN4_FD_EWP2_Cmd) -> [CAN4_FD_EWP2_Cmd]
  FDEWP3Cmd/1(CAN4_FD_EWP3_Cmd) -> [CAN4_FD_EWP3_Cmd]
  FDEXV1Cmd/1(CAN4_FD_EXV1_Cmd) -> [CAN4_FD_EXV1_Cmd]
  FDEXV2Cmd/1(CAN4_FD_EXV2_Cmd) -> [CAN4_FD_EXV2_Cmd]
  FDFWVCmd/1(CAN4_FD_FWV_Cmd) -> [CAN4_FD_FWV_Cmd]
  FDFrLeAPTCHeatPwrCmd/1(CAN4_FD_FrLeAPTCHeatPwr_Cmd) -> [CAN4_FD_FrLeAPTCHeatPwr_Cmd]
  FDFrRiAPTCHeatPwrCmd/1(CAN4_FD_FrRiAPTCHeatPwr_Cmd) -> [CAN4_FD_FrRiAPTCHeatPwr_Cmd]
  FDFrWPTCHeatPwrCmd/1(CAN4_FD_FrWPTCHeatPwr_Cmd) -> [CAN4_FD_FrWPTCHeatPwr_Cmd]
  FDRecyAutoCmd/1(CAN4_FD_RecyAuto_Cmd) -> [CAN4_FD_RecyAuto_Cmd]
  FDRrAPTCHeatPwrCmd/1(CAN4_FD_RrAPTCHeatPwr_Cmd) -> [CAN4_FD_RrAPTCHeatPwr_Cmd]
  FDSOTXVCmd/1(CAN4_FD_SOTXV_Cmd) -> [CAN4_FD_SOTXV_Cmd]
  FDSOV1Cmd/1(CAN4_FD_SOV1_Cmd) -> [CAN4_FD_SOV1_Cmd]
  FDSOV2Cmd/1(CAN4_FD_SOV2_Cmd) -> [CAN4_FD_SOV2_Cmd]
  FDSOV3Cmd/1(CAN4_FD_SOV3_Cmd) -> [CAN4_FD_SOV3_Cmd]
  FDTWVCmd/1(CAN4_FD_TWV_Cmd) -> [CAN4_FD_TWV_Cmd]
  FrCoolantflow/1(CAN4_Fr_Coolantflow) -> [CAN4_Fr_Coolantflow]
  FrCoolanttemp/1(CAN4_Fr_Coolanttemp) -> [CAN4_Fr_Coolanttemp]
  HPThermalRecoveryReq/1(CAN4_HPThermalRecoveryReq) -> [CAN4_HPThermalRecoveryReq]
  RrCoolantflow/1(CAN4_Rr_Coolantflow) -> [CAN4_Rr_Coolantflow]
  RrCoolanttemp/1(CAN4_Rr_Coolanttemp) -> [CAN4_Rr_Coolanttemp]
  sigAirIntenZon1St/1(CAN4_sigAirIntenZon1St) -> [CAN4_sigAirIntenZon1St]
  sigAirIntenZon3St/1(CAN4_sigAirIntenZon3St) -> [CAN4_sigAirIntenZon3St]
  sigAmbAirT/1(CAN4_sigAmbAirT) -> [CAN4_sigAmbAirT]
  sigCbnAirT/1(CAN4_sigCbnAirT) -> [CAN4_sigCbnAirT]
  sigCbnPTCPwrAct/1(CAN4_sigCbnPTCPwrAct) -> [CAN4_sigCbnPTCPwrAct]
  sigCbnSolarLeft/1(CAN4_sigCbnSolarLeft) -> [CAN4_sigCbnSolarLeft]
  sigCbnSolarRight/1(CAN4_sigCbnSolarRight) -> [CAN4_sigCbnSolarRight]
  sigClmtCmprPwrAct/1(CAN4_sigClmtCmprPwrAct) -> [CAN4_sigClmtCmprPwrAct]
  sigClntTHvBattOut/1(CAN4_sigClntTHvBattOut) -> [CAN4_sigClntTHvBattOut]
  sigDfrstSt/1(CAN4_sigDfrstSt) -> [CAN4_sigDfrstSt]
  sigHvacSt/1(CAN4_sigHvacSt) -> [CAN4_sigHvacSt]
  sigRecircSt/1(CAN4_sigRecircSt) -> [CAN4_sigRecircSt]
  sigSetTempZon1St/1(CAN4_sigSetTempZon1St) -> [CAN4_sigSetTempZon1St]
  sigSetTempZon2St/1(CAN4_sigSetTempZon2St) -> [CAN4_sigSetTempZon2St]
  sigSetTempZon3St/1(CAN4_sigSetTempZon3St) -> [CAN4_sigSetTempZon3St]
  sigWindDirZon1St/1(CAN4_sigWindDirZon1St) -> [CAN4_sigWindDirZon1St]
  sigWindDirZon3St/1(CAN4_sigWindDirZon3St) -> [CAN4_sigWindDirZon3St]
  bus_selector/1 -> ACSubMode/1(ACSubMode)  "<VOUTP_ACSubMode_enum>"
  [BOUTP_outputs] -> bus_selector/1
  Ground/1 -> APTCActFrRiPwr/1(APTCActFrRiPwr)
  Ground1/1 -> BatLoopActWtFlw/1(BatLoopActWtFlw)
  bus_selector1/1 -> BatteryMode/1(BatteryMode)  "<VOUTP_BatteryMode_enum>"
  [BOUTP_outputs] -> bus_selector1/1
  bus_selector2/1 -> CCUACLampSts/1(CCUACLampSts)  "<VOUTP_CCUACLampSts_flg>"
  [BOUTP_outputs] -> bus_selector2/1
  bus_selector3/1 -> CCUACMaxLampSts/1(CCUACMaxLampSts)  "<VOUTP_CCUACMaxLampSts_flg>"
  [BOUTP_outputs] -> bus_selector3/1
  bus_selector4/1 -> CCUAutoLampSts/1(CCUAutoLampSts)  "<VOUTP_CCUAutoLampSts_flg>"
  [BOUTP_outputs] -> bus_selector4/1
  Ground2/1 -> CCUAutoMidLampSts/1(CCUAutoMidLampSts)
  Ground3/1 -> CCUCbnPreACWkSts/1(CCUCbnPreACWkSts)
  Ground4/1 -> CCUCbnPreEstimdTi/1(CCUCbnPreEstimdTi)
  Ground5/1 -> CCUCbnPreSts/1(CCUCbnPreSts)
  Ground6/1 -> CCUDispalyRequest/1(CCUDispalyRequest)
  Ground7/1 -> CCUEcoSts/1(CCUEcoSts)
  Ground8/1 -> CCUFrtOnOffLampSts/1(CCUFrtOnOffLampSts)
  Ground9/1 -> CCUHEATMaxLampSts/1(CCUHEATMaxLampSts)
  Ground10/1 -> CCUHiVoltageReq/1(CCUHiVoltageReq)
  Ground11/1 -> CCURrOnOffLampSts/1(CCURrOnOffLampSts)
  bus_selector5/1 -> CCUSyncLampSts/1(CCUSyncLampSts)  "<VOUTP_CCUSyncLampSts_flg>"
  [BOUTP_outputs] -> bus_selector5/1
  bus_selector6/1 -> CabinMode/1(CabinMode)  "<VOUTP_CabinMode_enum>"
  [BOUTP_outputs] -> bus_selector6/1
  bus_selector7/1 -> CoolgFanActDuty/1(CoolgFanActDuty)  "<VOUTP_CoolgFanActDuty_pct>"
  [BOUTP_outputs] -> bus_selector7/1
  Ground12/1 -> DeiceModReq/1(DeiceModReq)
  bus_selector8/1 -> EDriveMode/1(EDriveMode)  "<VOUTP_EDriveMode_enum>"
  [BOUTP_outputs] -> bus_selector8/1
  bus_selector9/1 -> FDCTHCMCLEVentYSta/1(FDCTHCMCLEVentYSta)  "<VOUTP_FDCTHCCLEVentYSta_enum>"
  [BOUTP_outputs] -> bus_selector9/1
  bus_selector10/1 -> FDCTHCMCLEVentZSta/1(FDCTHCMCLEVentZSta)  "<VOUTP_FDCTHCCLEVentZSta_enum>"
  [BOUTP_outputs] -> bus_selector10/1
  bus_selector11/1 -> FDCTHCMCLVentSta/1(FDCTHCMCLVentSta)  "<VOUTP_FDCTHCCLVentENSta_flg>"
  [BOUTP_outputs] -> bus_selector11/1
  bus_selector12/1 -> FDCTHCMCREVentYSta/1(FDCTHCMCREVentYSta)  "<VOUTP_FDCTHCCREVentYSta_enum>"
  [BOUTP_outputs] -> bus_selector12/1
  bus_selector13/1 -> FDCTHCMCREVentZSta/1(FDCTHCMCREVentZSta)  "<VOUTP_FDCTHCCREVentZSta_enum>"
  [BOUTP_outputs] -> bus_selector13/1
  bus_selector23/1 -> FDAGSCmd/1(FDAGSCmd)  "<VOUTP_FDAGSCmd_enum>"
  [BOUTP_outputs] -> bus_selector23/1
  bus_selector24/1 -> FDBlowerCmd/1(FDBlowerCmd)  "<VOUTP_FDBlowerCmd_pct>"
  [BOUTP_outputs] -> bus_selector24/1
  bus_selector25/1 -> FDCompCmd/1(FDCompCmd)  "<VOUTP_FDCompCmd_rpm>"
  [BOUTP_outputs] -> bus_selector25/1
  bus_selector26/1 -> FDEWP1Cmd/1(FDEWP1Cmd)  "<VOUTP_FDEWP1Cmd_enum>"
  [BOUTP_outputs] -> bus_selector26/1
  bus_selector27/1 -> FDEWP2Cmd/1(FDEWP2Cmd)  "<VOUTP_FDEWP2Cmd_enum>"
  [BOUTP_outputs] -> bus_selector27/1
  bus_selector28/1 -> FDEWP3Cmd/1(FDEWP3Cmd)  "<VOUTP_FDEWP3Cmd_enum>"
  [BOUTP_outputs] -> bus_selector28/1
  bus_selector29/1 -> FDEXV1Cmd/1(FDEXV1Cmd)  "<VOUTP_FDEXV1Cmd_step>"
  [BOUTP_outputs] -> bus_selector29/1
  bus_selector30/1 -> FDEXV2Cmd/1(FDEXV2Cmd)  "<VOUTP_FDEXV2Cmd_step>"
  [BOUTP_outputs] -> bus_selector30/1
  bus_selector31/1 -> FDFWVCmd/1(FDFWVCmd)  "<VOUTP_FDFWVCmd_flg>"
  [BOUTP_outputs] -> bus_selector31/1
  bus_selector32/1 -> FDFrLeAPTCHeatPwrCmd/1(FDFrLeAPTCHeatPwrCmd)  "<VOUTP_FDFrLeAPTCHeatPwrCmd_W>"
  [BOUTP_outputs] -> bus_selector32/1
  bus_selector33/1 -> FDFrRiAPTCHeatPwrCmd/1(FDFrRiAPTCHeatPwrCmd)  "<VOUTP_FDFrRiAPTCHeatPwrCmd_W>"
  [BOUTP_outputs] -> bus_selector33/1
  bus_selector34/1 -> FDFrWPTCHeatPwrCmd/1(FDFrWPTCHeatPwrCmd)  "<VOUTP_FDFrWPTCHeatPwrCmd_W>"
  [BOUTP_outputs] -> bus_selector34/1
  bus_selector35/1 -> FDRecyAutoCmd/1(FDRecyAutoCmd)  "<VOUTP_FDRecyAutoCmd_enum>"
  [BOUTP_outputs] -> bus_selector35/1
  bus_selector36/1 -> FDRrAPTCHeatPwrCmd/1(FDRrAPTCHeatPwrCmd)  "<VOUTP_FDRrAPTCHeatPwrCmd_W>"
  [BOUTP_outputs] -> bus_selector36/1
  bus_selector37/1 -> FDSOTXVCmd/1(FDSOTXVCmd)  "<VOUTP_FDSOTXVCmd_flg>"
  [BOUTP_outputs] -> bus_selector37/1
  bus_selector38/1 -> FDSOV1Cmd/1(FDSOV1Cmd)  "<VOUTP_FDSOV1Cmd_flg>"
  [BOUTP_outputs] -> bus_selector38/1
  bus_selector39/1 -> FDSOV2Cmd/1(FDSOV2Cmd)  "<VOUTP_FDSOV2Cmd_flg>"
  [BOUTP_outputs] -> bus_selector39/1
  bus_selector40/1 -> FDSOV3Cmd/1(FDSOV3Cmd)  "<VOUTP_FDSOV3Cmd_flg>"
  [BOUTP_outputs] -> bus_selector40/1
  bus_selector41/1 -> FDTWVCmd/1(FDTWVCmd)  "<VOUTP_FDTWVCmd_pct>"
  [BOUTP_outputs] -> bus_selector41/1
  Ground13/1 -> FrCoolantflow/1(FrCoolantflow)
  Ground14/1 -> FrCoolanttemp/1(FrCoolanttemp)
  Ground15/1 -> HPThermalRecoveryReq/1(HPThermalRecoveryReq)
  Ground16/1 -> RrCoolantflow/1(RrCoolantflow)
  Ground17/1 -> RrCoolanttemp/1(RrCoolanttemp)
  bus_selector42/1 -> sigAirIntenZon1St/1(sigAirIntenZon1St)  "<VOUTP_sigAirIntenZon1St_enum>"
  [BOUTP_outputs] -> bus_selector42/1
  Ground18/1 -> sigAirIntenZon3St/1(sigAirIntenZon3St)
  bus_selector43/1 -> sigAmbAirT/1(sigAmbAirT)  "<VOUTP_sigAmbAirT_C>"
  [BOUTP_outputs] -> bus_selector43/1
  bus_selector44/1 -> sigCbnAirT/1(sigCbnAirT)  "<VOUTP_sigCbnAirT_C>"
  [BOUTP_outputs] -> bus_selector44/1
  bus_selector45/1 -> sigCbnSolarLeft/1(sigCbnSolarLeft)  "<VOUTP_sigCbnSolarLeft_W>"
  [BOUTP_outputs] -> bus_selector45/1
  bus_selector46/1 -> sigCbnSolarRight/1(sigCbnSolarRight)  "<VOUTP_sigCbnSolarRight_W>"
  [BOUTP_outputs] -> bus_selector46/1
  Ground20/1 -> sigClmtCmprPwrAct/1(sigClmtCmprPwrAct)
  bus_selector47/1 -> sigClntTHvBattOut/1(sigClntTHvBattOut)  "<VOUTP_sigClntTHvBattOut_C>"
  [BOUTP_outputs] -> bus_selector47/1
  bus_selector48/1 -> sigDfrstSt/1(sigDfrstSt)  "<VOUTP_sigDfrstSt_flg>"
  [BOUTP_outputs] -> bus_selector48/1
  Ground21/1 -> sigHvacSt/1(sigHvacSt)
  bus_selector49/1 -> sigRecircSt/1(sigRecircSt)  "<VOUTP_sigRecircSt_flg>"
  [BOUTP_outputs] -> bus_selector49/1
  bus_selector50/1 -> sigSetTempZon1St/1(sigSetTempZon1St)  "<VOUTP_sigSetTempZon1St_C>"
  [BOUTP_outputs] -> bus_selector50/1
  bus_selector51/1 -> sigSetTempZon2St/1(sigSetTempZon2St)  "<VOUTP_sigSetTempZon2St_C>"
  [BOUTP_outputs] -> bus_selector51/1
  Ground22/1 -> sigSetTempZon3St/1(sigSetTempZon3St)
  bus_selector52/1 -> sigWindDirZon1St/1(sigWindDirZon1St)  "<VOUTP_sigWindDirZon1St_enum>"
  [BOUTP_outputs] -> bus_selector52/1
  Ground23/1 -> sigWindDirZon3St/1(sigWindDirZon3St)
  [BOUTP_outputs] -> bus_selector53/1
  bus_selector53/1 -> sigCbnPTCPwrAct/1(sigCbnPTCPwrAct)  "<VOUTP_sigCbnPTCPwrAct_W>"
  [BOUTP_outputs] -> bus_selector17/1
  bus_selector17/1 -> FDCTHCMDrVentSta/1(FDCTHCMDrVentSta)  "<VOUTP_FDCTHCRVentENSta_flg>"
  bus_selector14/1 -> FDCTHCMCRVentSta/1(FDCTHCMCRVentSta)  "<VOUTP_FDCTHCLEVentModeSta_enum>"
  [BOUTP_outputs] -> bus_selector15/1
  bus_selector18/1 -> FDCTHCMDrEVentZSta/1(FDCTHCMDrEVentZSta)  "<VOUTP_FDCTHCLVentENSta_flg>"
  [BOUTP_outputs] -> bus_selector14/1
  bus_selector15/1 -> FDCTHCMDrEVentModeSta/1(FDCTHCMDrEVentModeSta)  "<VOUTP_FDCTHCLEVentYSta_enum>"
  [BOUTP_outputs] -> bus_selector18/1
  bus_selector16/1 -> FDCTHCMDrEVentYSta/1(FDCTHCMDrEVentYSta)  "<VOUTP_FDCTHCLEVentZSta_enum>"
  [BOUTP_outputs] -> bus_selector16/1
  bus_selector21/1 -> FDCTHCMPsEVentZSta/1(FDCTHCMPsEVentZSta)  "<VOUTP_FDCTHCREVentZSta_enum>"
  [BOUTP_outputs] -> bus_selector22/1
  [BOUTP_outputs] -> bus_selector21/1
  bus_selector19/1 -> FDCTHCMPsEVentModeSta/1(FDCTHCMPsEVentModeSta)  "<VOUTP_FDCTHCREVentModeSta_enum>"
  [BOUTP_outputs] -> bus_selector20/1
  [BOUTP_outputs] -> bus_selector19/1
  bus_selector20/1 -> FDCTHCMPsEVentYSta/1(FDCTHCMPsEVentYSta)  "<VOUTP_FDCTHCREVentYSta_enum>"
  bus_selector22/1 -> FDCTHCMPsVentSta/1(FDCTHCMPsVentSta)  "<VOUTP_FDCTHCRVentENSta_flg>"
